simulink model "Example5"  (Simulink 6.0)
settings: Solver=ode45  StartTime=0.0  StopTime=10.0  RelTol=1e-3
settings Model: LastModifiedBy=Administrator

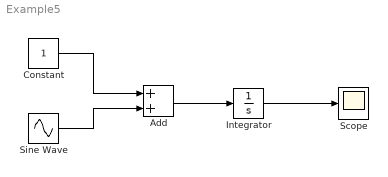
== system Example5 ==
  Add : Sum  OutScaling=2^-10
  Constant : Constant
  Integrator : Integrator
  Scope : Scope
  Sine Wave : Sin  SampleTime=0
  wires:
  Constant/1 -> Add/1
  Sine Wave/1 -> Add/2
  Add/1 -> Integrator/1
  Integrator/1 -> Scope/1
